simulink library "ammclib_bam_S32K3xx"  (R2016a)
(part 21 of 50)

      |         if f32CC2sc>2^31-1
      |           f32CC2sc=2^31-1;
      |           warning(['Parameter f32CC2sc of ' gcb ' exceeds the fixed-point range.']);
      |         end
      |         if f32CC2sc<-2^31
      |           f32CC2sc=-2^31;
      |           warning(['Parameter f32CC2sc of ' gcb ' exceeds the fixed-point range.']);
      |         end
      |         f32LowerLimit=-2147483648;
      |         f32UpperLimit=2147483647;
      |         c1f=SampleTime*0.5*wmax/3.141592653589793;
      |         u16NShiftI=ceil(log2(abs(c1f)));
      |         if u16NShiftI<0
      |           u16NShiftI=0;
      |         end
      |         if u16NShiftI>31
      |           u16NShiftI=31;
      |           warning(['Parameter u16NShiftI of ' gcb ' exceeds the fixed-point range.']);
      |         end
      |         f32C1=round(c1f*2^(-u16NShiftI)*2^31);
      |         if f32C1>2^31-1
      |           f32C1=2^31-1;
      |           warning(['Parameter f32C1 of ' gcb ' exceeds the fixed-point range.']);
      |         end
      |         if f32C1<-2^31
      |           f32C1=-2^31;
      |           warning(['Parameter f32C1 of ' gcb ' exceeds the fixed-point range.']);
      |         end
      |         if isnan(f32ADCMaxError)
      |           if ~strcmp(f32ADCMaxError_bkup,'0')
      |             set_param(gcb,'f32ADCMaxError','0');
      |           end
      |         else
      |           tmps=num2str(f32ADCMaxError);
      |           if ~strcmp(f32ADCMaxError_bkup,tmps)
      |             set_param(gcb,'f32ADCMaxError',tmps);
      |           end
      |         end
      |         if isnan(f32CC1sc)
      |           if ~strcmp(f32CC1sc_bkup,'0')
      |             set_param(gcb,'f32CC1sc','0');
      |           end
      |         else
      |           tmps=num2str(f32CC1sc);
      |           if ~strcmp(f32CC1sc_bkup,tmps)
      |             set_param(gcb,'f32CC1sc',tmps);
      |           end
      |         end
      |         if isnan(f32CC2sc)
      |           if ~strcmp(f32CC2sc_bkup,'0')
      |             set_param(gcb,'f32CC2sc','0');
      |           end
      |         else
      |           tmps=num2str(f32CC2sc);
      |           if ~strcmp(f32CC2sc_bkup,tmps)
      |             set_param(gcb,'f32CC2sc',tmps);
      |           end
      |         end
      |         if isnan(f32UpperLimit)
      |           if ~strcmp(f32UpperLimit_bkup,'0')
      |             set_param(gcb,'f32UpperLimit','0');
      |           end
      |         else
      |           tmps=num2str(f32UpperLimit);
      |           if ~strcmp(f32UpperLimit_bkup,tmps)
      |             set_param(gcb,'f32UpperLimit',tmps);
      |           end
      |         end
      |         if isnan(f32LowerLimit)
      |           if ~strcmp(f32LowerLimit_bkup,'0')
      |             set_param(gcb,'f32LowerLimit','0');
      |           end
      |         else
      |           tmps=num2str(f32LowerLimit);
      |           if ~strcmp(f32LowerLimit_bkup,tmps)
      |             set_param(gcb,'f32LowerLimit',tmps);
      |           end
      |         end
      |         if isnan(u16NShiftPI)
      |           if ~strcmp(u16NShiftPI_bkup,'0')
      |             set_param(gcb,'u16NShiftPI','0');
      |           end
      |         else
      |           tmps=num2str(u16NShiftPI);
      |           if ~strcmp(u16NShiftPI_bkup,tmps)
      |             set_param(gcb,'u16NShiftPI',tmps);
      |           end
      |         end
      |         if isnan(f32C1)
      |           if ~strcmp(f32C1_bkup,'0')
      |             set_param(gcb,'f32C1','0');
      |           end
      |         else
      |           tmps=num2str(f32C1);
      |           if ~strcmp(f32C1_bkup,tmps)
      |             set_param(gcb,'f32C1',tmps);
      |           end
      |         end
      |         if isnan(u16NShiftI)
      |           if ~strcmp(u16NShiftI_bkup,'0')
      |             set_param(gcb,'u16NShiftI','0');
      |           end
      |         else
      |           tmps=num2str(u16NShiftI);
      |           if ~strcmp(u16NShiftI_bkup,tmps)
      |             set_param(gcb,'u16NShiftI',tmps);
      |           end
      |         end
      |       end
      |     end
      |   catch
      |    warning(['Sample time cannot be calculated for the block ' gcb])
      |   end
      | end
      mask DialogControl timeHint Prompt: Note: Implementation parameters cannot be calculated yet because the block's inherited sample time is unknown. Simulink will update the sample time when you run the simulation.
      mask Display:
      | color('black');
      | pos = get_param(gcb, 'Position');
      | width = pos(3) - pos(1);
      | height = pos(4) - pos(2);
      | tX=width/2;
      | tY=height - 8;
      | color('black');
      | text(tX,tY, 'AMCLIB_Windmilling_F32', 'horizontalAlignment', 'center');
      | if showStates == 2
      |   color('red');
      |   text(tX,tY - 20, ['debugging mode' char(13) char(10) '(limited performance)'], 'horizontalAlignment', 'center');
      | end
